simulink model "BIO_csi_sf"  (R2017a)
settings: Solver=ode4  StartTime=0.0  StopTime=6  FixedStep=1e-4  RelTol=1e-3
InitFcn:
  | SimulinkInit
values from neighbouring files (symbols this model uses):
  L1 = 40e-3    (= 0.04)    [pruebauGridSF.m]
  R1 = 0.1    [pruebauGridSF.m]
libraries: dsparch4 x2, mpclib x1
settings Model: Creator=carma  LastModifiedBy=carma
settings OptimizationCC: DefaultParameterBehavior=Inlined  PassReuseOutputArgsAs=Individual arguments
settings DebuggingCC: ParameterTunabilityLossMsg=error
settings SFSimCC: MATLABDynamicMemAlloc=off
settings RTWCC: SystemTargetFile=ert.tlc  TemplateMakefile=ert_default_tmf  Description=Embedded Coder  GenerateReport=on  IncludeHyperlinkInReport=on  LaunchReport=on  GenerateTraceInfo=on  GenerateTraceReport=on  GenerateTraceReportSl=on  GenerateTraceReportSf=on  GenerateTraceReportEml=on
settings CodeAppCC: ForceParamTrailComments=on  IgnoreCustomStorageClasses=off  OperatorAnnotations=on  SimulinkDataObjDesc=on  SFDataObjDesc=on  MATLABFcnDesc=on  InsertBlockDesc=on  MATLABSourceComments=on
settings ERTTargetCC: TargetLangStandard=C99 (ISO)  GenerateSampleERTMain=on  SupportContinuousTime=on  InlinedParameterPlacement=NonHierarchical  ERTCustomFileTemplate=example_file_process.tlc

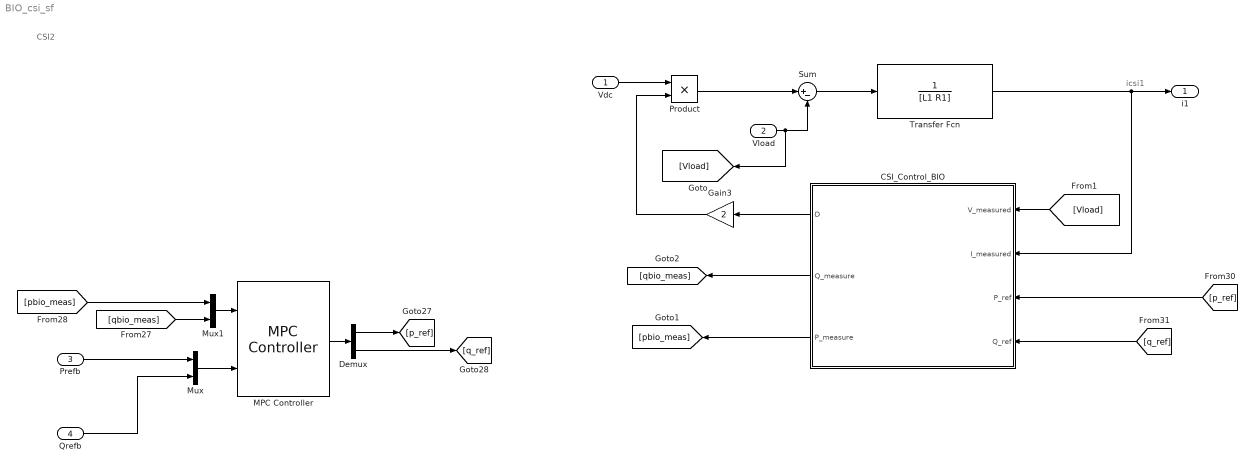
== system BIO_csi_sf ==
  note: CSI2
  note: icsi1
  Vdc : Inport
  Vload : Inport  Port=2
  Prefb : Inport  Port=3
  Qrefb : Inport  Port=4
  CSI_Control_BIO : Subsystem  mask{A=[0.0201   -0.039932     0.01986], B=[1     -1.9966       0.998], T=0.0001, st_time=.1, Dn=[1     -1.0364], Dd=[1    -0.96364]}
      mask prompts: A "Numerador del control PR(z)"; B "Denominador del control PR(z)"; T "Tiempo de muestreo"; st_time "Tiempo_muerto"; Dn "Dn (Numerador de D(z))"; Dd "Dd (numerador de D(z))"
      mask DialogControl descripcion Prompt: Lazo de control de corriente para inversor monofasico. La entrada es un setpoint de potencia [P, Q]. Con ese setpoint se calcula la referencia de corriente sinusoidal deacuerdo a la tension medida de la red. Por lo anterior este controlador solo es valido para un inversor conectado a la red pues hara que se comporte como un CSI.
      mask DialogControl Control2 Prompt: Dn y Dd corresponden al numerador y denominador de la funcion de transferencia en Z (denominada D(z)) que hara un desfase de 90 de las señales medidas de tension y corriente del inversor. Estos desfases permiten mimificar las señales alfa y beta, de esta forma usar la misma teoria de potencia instantanea para el caso monofasico.
  Demux : Demux  Outputs=2
  Gain3 : Gain  Gain=2
  MPC Controller : mpclib/MPC Controller  mpcobj=mpcobj  x0=[]  is_multiple=0  enable_value=0  return_u0=off  ref_from_ws=off  ref_signal_name=[]  ref_preview=on  md_from_ws=off  md_signal_name=[]  md_preview=on  from_project=off  project_file=MPCtask.mat  md_inport=off  mv_inport=off  cost_outport=off  return_sequence=off  return_qpstatus=off  return_state=off  state_inport=off  lims_inport=off  ywt_inport=off  is_designfromscratch=0  uwt_inport=off  duwt_inport=off  rhoeps_inport=off  uref_inport=off  n_ts=0.1  n_mv=2  n_md=0  n_ud=0  n_mo=2  n_uo=0  BlockDataType=double  SampleTimeInherited=off  switch_inport=off
  Mux : Mux  Inputs=2
  Mux1 : Mux  Inputs=2
  Product : Product
  Sum : Sum  Inputs=|+-
  Transfer Fcn : TransferFcn  Denominator=[L1 R1]
  i1 : Outport
  wires:
  Sum/1 -> Transfer Fcn/1
  Vload/1 -> [Vload], Sum/2
  Product/1 -> Sum/1
  Gain3/1 -> Product/2
  CSI_Control_BIO/2(Q_measure) -> [qbio_meas]
  Transfer Fcn/1 -> i1/1, CSI_Control_BIO/2(I_measured)
  [Vload] -> CSI_Control_BIO/1(V_measured)
  CSI_Control_BIO/1(D) -> Gain3/1
  [pbio_meas] -> Mux1/1
  [qbio_meas] -> Mux1/2
  MPC Controller/1 -> Demux/1
  Mux1/1 -> MPC Controller/1
  Demux/2 -> [q_ref]
  Mux/1 -> MPC Controller/2
  Demux/1 -> [p_ref]
  Prefb/1 -> Mux/1
  Qrefb/1 -> Mux/2
  CSI_Control_BIO/3(P_measure) -> [pbio_meas]
  [p_ref] -> CSI_Control_BIO/3(P_ref)
  [q_ref] -> CSI_Control_BIO/4(Q_ref)
  Vdc/1 -> Product/1

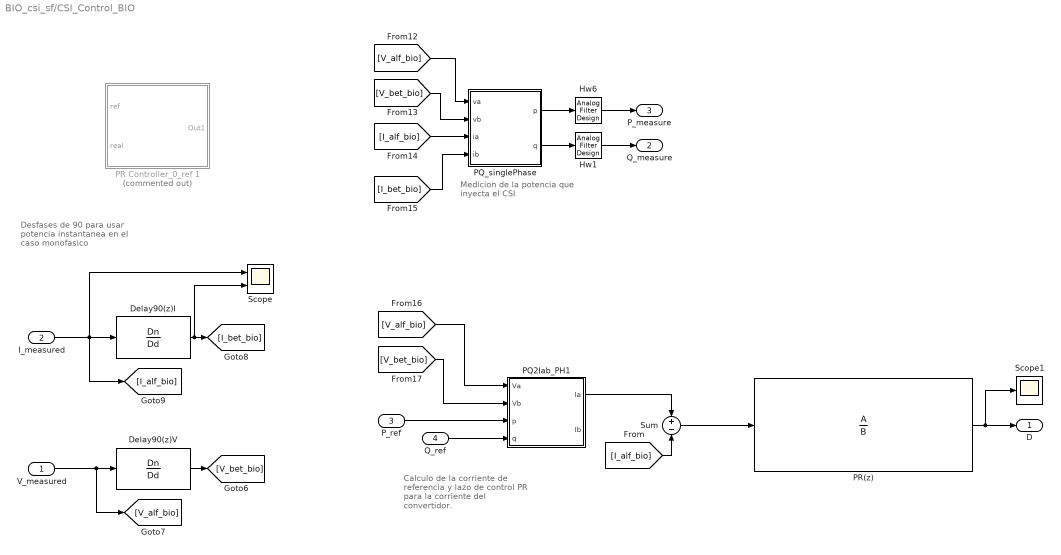
== system BIO_csi_sf/CSI_Control_BIO ==
  note: Medicion de la potencia que inyecta el CSI
  note: Desfases de 90 para usar potencia
      | instantanea en el caso monofasico
  note: Calculo de la corriente de referencia
      | y lazo de control PR para la corriente
      | del convertidor.
  V_measured : Inport
  I_measured : Inport  Port=2
  P_ref : Inport  Port=3
  Q_ref : Inport  Port=4
  Delay90(z)I : DiscreteTransferFcn  Numerator=Dn  Denominator=Dd  SampleTime=T
  Delay90(z)V : DiscreteTransferFcn  Numerator=Dn  Denominator=Dd  SampleTime=T
  Hw1 : dsparch4/Analog Filter Design  method=Bessel  filttype=Lowpass  N=4  Wlo=30*2*pi  Whi=80  Rp=2  Rs=80
  Hw6 : dsparch4/Analog Filter Design  method=Bessel  filttype=Lowpass  N=4  Wlo=30*2*pi  Whi=80  Rp=2  Rs=80
  PQ2Iab_PH1 : MATLAB Function  TreatAsAtomicUnit=on
  PQ_singlePhase : MATLAB Function  TreatAsAtomicUnit=on
  PR Controller_0_ref 1 : Subsystem  Commented=on  mask{Kp=40/100, Ki=200, wa=2, w0=60*2*pi, st_time=1e-3}
      mask prompts: Kp "Ganancia Proporcional"; Ki "Ganancia Integral"; wa "Ancho camapana resonancia"; w0 "Frecuencia Central"; st_time "Tiempo muerto (Start)"
      mask Display:
      | port_label('input',1,'ref')
      | port_label('input',2,'sens')
      | port_label('output',1,'out')
      | 
      | plot(.4+[0:.01:pi/10], .32+sin(40*[0:.01:pi/10])/13)
      | 
      | plot([.4 .6],.05+[.5 .7])
      | plot([.4 .6],.05+[.9 .7])
      | plot([.4 .4],.05+[.9 .5])
      | 
      | text(.27,.37,'\fontsize{25} \int', 'texmode', 'on')
  PR(z) : DiscreteTransferFcn  Numerator=A  Denominator=B  SampleTime=T
  Scope : Scope  NumInputPorts=2
  Scope1 : Scope
  Sum : Sum  Inputs=+-
  D : Outport
  Q_measure : Outport  Port=2
  P_measure : Outport  Port=3
  wires:
  I_measured/1 -> Scope/1, Delay90(z)I/1, [I_alf_bio]
  PQ_singlePhase/2(q) -> Hw1/1
  [V_bet_bio] -> PQ2Iab_PH1/2(Vb)
  Delay90(z)I/1 -> Scope/2, [I_bet_bio]
  [I_bet_bio] -> PQ_singlePhase/4(ib)
  [I_alf_bio] -> PQ_singlePhase/3(ia)
  [V_alf_bio] -> PQ2Iab_PH1/1(Va)
  PQ_singlePhase/1(p) -> Hw6/1
  Delay90(z)V/1 -> [V_bet_bio]
  [V_bet_bio] -> PQ_singlePhase/2(vb)
  [V_alf_bio] -> PQ_singlePhase/1(va)
  V_measured/1 -> Delay90(z)V/1, [V_alf_bio]
  P_ref/1 -> PQ2Iab_PH1/3(p)
  Q_ref/1 -> PQ2Iab_PH1/4(q)
  Sum/1 -> PR(z)/1
  [I_alf_bio] -> Sum/2
  PQ2Iab_PH1/1(Ia) -> Sum/1
  PR(z)/1 -> Scope1/1, D/1
  Hw6/1 -> P_measure/1
  Hw1/1 -> Q_measure/1

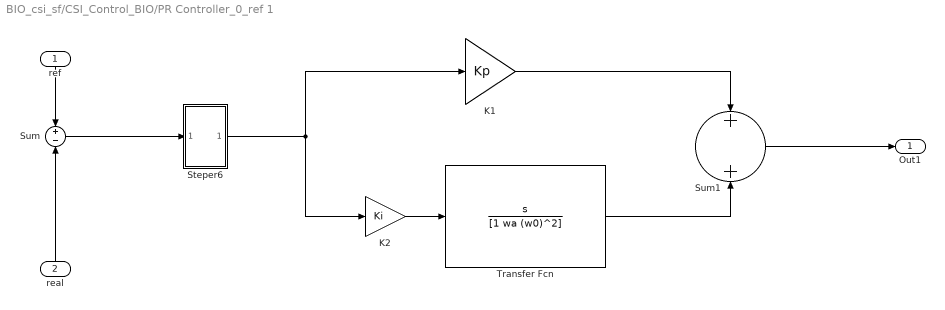
== system BIO_csi_sf/CSI_Control_BIO/PR Controller_0_ref 1 ==
  ref : Inport
  real : Inport  Port=2
  K1 : Gain  Gain=Kp
  K2 : Gain  Gain=Ki
  Steper6 : Subsystem
  Sum : Sum  Inputs=+-
  Sum1 : Sum  Inputs=+|+
  Transfer Fcn : TransferFcn  Numerator=[1 0]  Denominator=[1 wa (w0)^2]
  Out1 : Outport
  wires:
  real/1 -> Sum/2
  ref/1 -> Sum/1
  Sum/1 -> Steper6/1(In1)
  K1/1 -> Sum1/1
  Transfer Fcn/1 -> Sum1/2
  K2/1 -> Transfer Fcn/1
  Steper6/1(Out1) -> K1/1, K2/1
  Sum1/1 -> Out1/1

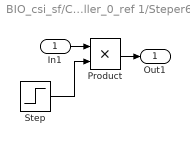
== system BIO_csi_sf/CSI_Control_BIO/PR Controller_0_ref 1/Steper6 ==
  In1 : Inport
  Product : Product
  Step : Step  Time=st_time  SampleTime=0
  Out1 : Outport
  wires:
  Product/1 -> Out1/1
  In1/1 -> Product/1
  Step/1 -> Product/2

== matlab function BIO_csi_sf/CSI_Control_BIO/PQ_singlePhase ==
  data: va input; p output; vb input; ia input; ib input; q output
function [p, q] = fcn(va, vb, ia, ib)
% Esta funcion calcula la potencia activa y reactiva instantanea
% para el caso mnosofasico. En la revision de 2 papers he observado
% que una manera de extender la teoria de potencia al caso monofasico
% es asumiendo la tension o corriente de una fase como la componente
% alpha y hacer un desfase de 90 grados para obtener una version
% artificial de beta.

paux=va*ia+vb*ib;
if(paux > 20e4)
    paux = 20e4;
end
if(paux < -20e4)
    paux = -20e-4;
end

p = paux/2; % potencia activa instantanea

qaux = vb*ia-va*ib;

if(qaux>20e4)
    qaux=20e4;
end
if(qaux<-20e4)
    qaux=-20e4;
end

q = qaux/2; % potencia reactiva instantanea

== matlab function BIO_csi_sf/CSI_Control_BIO/PQ2Iab_PH1 ==
  data: Va input; Ia output; Vb input; p input; q input; Ib output
function [Ia, Ib] = fcn(Va, Vb, p, q)
%#codegen

% divide by zero protection
if(abs((Va^2+Vb^2))<=1000*eps(0))
    det = 1/eps(0);
else
    det = 1/(Va^2+Vb^2); % constante auxiliar
end;
%det = 1/(Va^2+Vb^2);

Mat = det*[Va Vb; Vb -Va];
Iab = Mat*[2*p;2*q];

Iaaux = Iab(1);
Ibaux = Iab(2);

ilim=1e3;

if(Iaaux>ilim)
    Iaaux=ilim;
end;
if(Iaaux<-ilim)
    Iaaux =-ilim;    
end;

if(isnan(Iaaux))
    Iaaux=0;
end;
%-----------------


if(Ibaux>ilim)
    Ibaux=ilim;
end;
if(Ibaux<-ilim)
    Ibaux =-ilim;    
end;

if(isnan(Ibaux))
    Ibaux=0;
end;
%-----------------


Ia = Iaaux;
Ib = Ibaux;
